simulink model "dc_motor_torque_model"  (R2019a)
settings: Solver=VariableStepAuto  StartTime=0.0  StopTime=50.0  RelTol=1e-3
values from neighbouring files (symbols this model uses):
  J = 0.010    (= 0.01)    [dc_motor_simulink_modelling.m]
  K_e = 0.24+0.0080    (= 0.248)    [dc_motor_simulink_modelling.m]
  K_t = 0.36    [dc_motor_simulink_modelling.m]
  L = 1    [dc_motor_simulink_modelling.m]
  m3 = 0.00215055254478    [data_workspace.mat]    (also in p.m = constant3(1))
  m4 = 0.000906699781425    [data_workspace.mat]    (also in p.m = constant4(1))
  m_p1 = 0.00317019595645    [data_workspace.mat]    (also in p.m = constant_p1(1))
  m_p2 = 0.00218886821705    [data_workspace.mat]    (also in p.m = constant_p2(1))
  m_p3 = 0.00103611475607    [data_workspace.mat]    (also in p.m = constant_p3(1))
  pinion_radius = 0.175    [dc_motor_simulink_modelling.m]
  rd = (pi/30)    (= 0.10471975512)    [dc_motor_simulink_modelling.m]
settings Model: Creator=fotoyis  LastModifiedBy=fotoyis

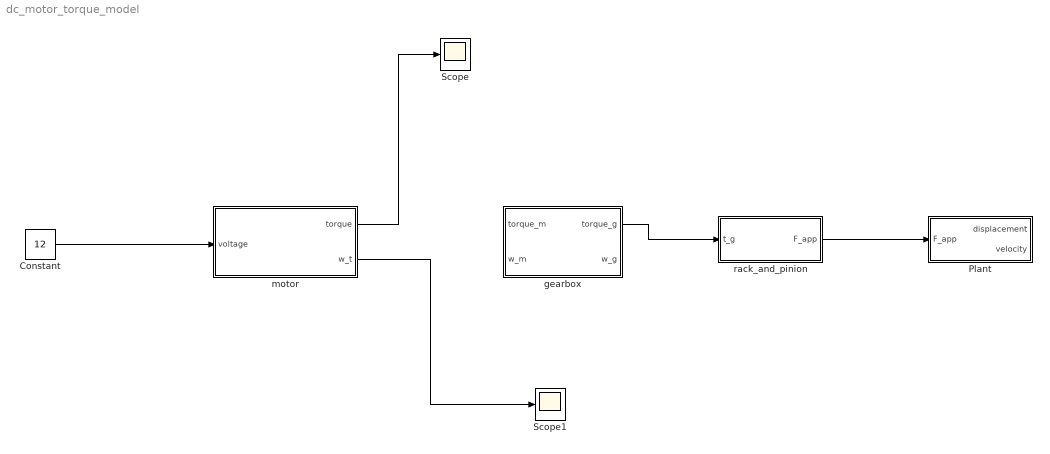
== system dc_motor_torque_model ==
  Constant : Constant  Value=12
  Plant : Subsystem
  Scope : Scope
  Scope1 : Scope
  gearbox : Subsystem
  motor : Subsystem
  rack_and_pinion : Subsystem
  wires:
  gearbox/1(torque_g) -> rack_and_pinion/1(t_g)
  rack_and_pinion/1(F_app) -> Plant/1(F_app)
  Constant/1 -> motor/1(voltage)
  motor/1(torque) -> Scope/1
  motor/2(w_t) -> Scope1/1

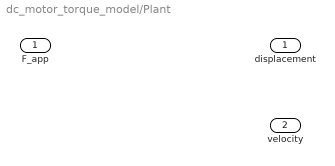
== system dc_motor_torque_model/Plant ==
  F_app : Inport
  displacement : Outport
  velocity : Outport  Port=2

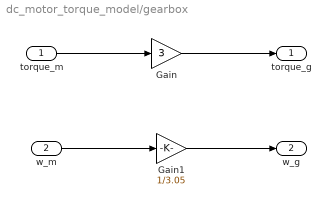
== system dc_motor_torque_model/gearbox ==
  "torque_m " : Inport
  w_m : Inport  Port=2
  Gain : Gain  Gain=3
  Gain1 : Gain  Gain=1/3.05
  torque_g : Outport
  w_g : Outport  Port=2
  wires:
  "torque_m "/1 -> Gain/1
  Gain/1 -> torque_g/1
  w_m/1 -> Gain1/1
  Gain1/1 -> w_g/1

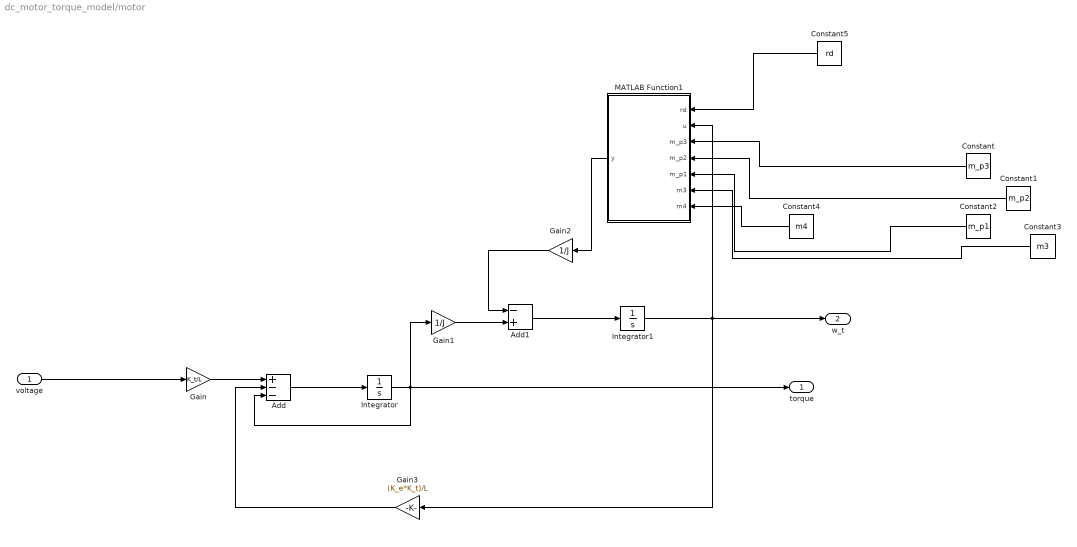
== system dc_motor_torque_model/motor ==
  voltage : Inport
  Add : Sum  Inputs=+--
  Add1 : Sum  Inputs=-+
  Constant : Constant  Value=m_p3
  Constant1 : Constant  Value=m_p2
  Constant2 : Constant  Value=m_p1
  Constant3 : Constant  Value=m3
  Constant4 : Constant  Value=m4
  Constant5 : Constant  Value=rd
  Gain : Gain  Gain=K_t/L
  Gain1 : Gain  Gain=1/J
  Gain2 : Gain  Gain=1/J
  Gain3 : Gain  Gain=(K_e*K_t)/L
  Integrator : Integrator
  Integrator1 : Integrator
  MATLAB Function1 : MATLAB Function  TreatAsAtomicUnit=on
  torque : Outport
  w_t : Outport  Port=2
  wires:
  Gain/1 -> Add/1
  voltage/1 -> Gain/1
  Gain3/1 -> Add/2
  Add/1 -> Integrator/1
  Gain1/1 -> Add1/2
  Gain2/1 -> Add1/1
  Integrator/1 -> Add/3, torque/1, Gain1/1
  Add1/1 -> Integrator1/1
  Constant1/1 -> MATLAB Function1/4(m_p2)
  MATLAB Function1/1(y) -> Gain2/1
  Constant3/1 -> MATLAB Function1/6(m3)
  Constant2/1 -> MATLAB Function1/5(m_p1)
  Constant/1 -> MATLAB Function1/3(m_p3)
  Constant4/1 -> MATLAB Function1/7(m4)
  Integrator1/1 -> MATLAB Function1/2(u), w_t/1, Gain3/1
  Constant5/1 -> MATLAB Function1/1(rd)

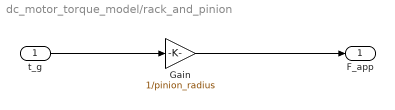
== system dc_motor_torque_model/rack_and_pinion ==
  t_g : Inport
  Gain : Gain  Gain=1/pinion_radius
  F_app : Outport
  wires:
  Gain/1 -> F_app/1
  t_g/1 -> Gain/1

== matlab function dc_motor_torque_model/motor/MATLAB Function1 ==
  data: rd input; u input; y output; m_p3 input; m_p2 input; m_p1 input; m3 input; m4 input
function y = fcn(rd, u,m_p3,m_p2,m_p1,m3, m4)
    y_ = 0;
     if((u >-150*rd)&&(u<-95*rd))
         y_ = m_p3*u-0.4801;
     elseif((u>-91*rd)&&(u<-74*rd))
         y_ =  m_p2*u-0.362;
             
     elseif((u>-71*rd)&&(u<-43*rd))
          y_ = m_p1*u-0.2877;
             
     elseif((u > 40*rd)&&(u <= 91*rd))
          y_ =  m3*u + 0.3271;
              
     elseif((u >91*rd)&&(u < 180*rd))
                  
          y_ =  m4*u + 0.4486;
     end
     
y = y_;
